simulink model "TwoSignal_RedisConnect"  (R2024a)
settings: Solver=VariableStepAuto  StartTime=0.0  StopTime=10.0  RelTol=1e-3
settings Model: Creator=deshazere  LastModifiedBy=deshazere

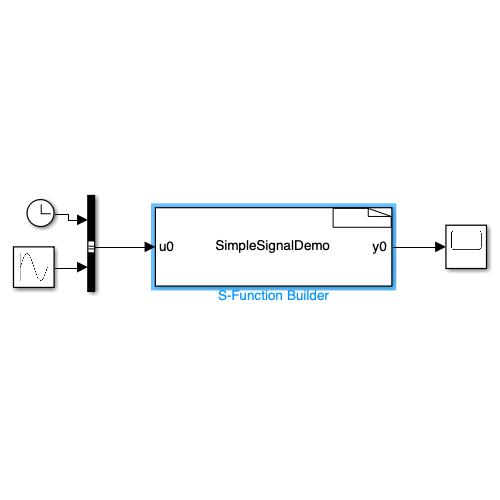
[thumbnail: Simulink's stored preview of the top-level diagram]
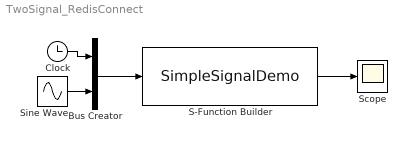
== system TwoSignal_RedisConnect ==
  Bus Creator : BusCreator  Inputs=2
  Clock : Clock
  S-Function Builder : S-Function  FunctionName=SimpleSignalDemo  SFunctionModules=SimpleSignalDemo_wrapper.c  SFunctionDeploymentMode=off  EnableBusSupport=off  mask(S-Function Builder){}
      mask help: Simulink:masks:SFunctionBuilder_MD
      mask init:
      | val = [[.9  0.75 0.75 1 1 .9 .9 1]',[1 1 0.75 0.75 .9 .9 1 .9]'];try , sys = get_param(gcb,'SfunBuilderFcnName');if isempty(sys), sys = get_param(gcb,'FunctionName'); end,catch, sys = get_param(gcb,'FunctionName'); end
      settings: CopyFcn=set_param(gcbh,'LinkStatus','none')  OpenFcn=sfunctionwizard(gcbh)
      mask Display:
      | plot(val(:,1),val(:,2))
      | disp(sys)
      | port_label('input',1,sprintf('%s', 'u0'),'interpreter','tex')
      | port_label('output',1,sprintf('%s', 'y0'),'interpreter','tex')
  Scope : Scope
  Sine Wave : Sin  SampleTime=0
  wires:
  S-Function Builder/1 -> Scope/1
  Sine Wave/1 -> Bus Creator/2
  Bus Creator/1 -> S-Function Builder/1
  Clock/1 -> Bus Creator/1
